simulink model "diva_R2020a"  (R2020a)
settings: Solver=FixedStepDiscrete  StartTime=0.0  StopTime=0.66  RelTol=1e-3  EnableMultiTasking=on
InitFcn:
  | diva_callback_initfcn
StopFcn:
  | diva_callback_stopfcn
undefined symbols (not defined in the file or in its folder): diva_hanning
libraries: simulink x13
CloseFcn:
  | diva_callback_closefcn
settings Model: Creator=alfnie  LastModifiedBy=alfnie
settings DataIOCC: SaveFormat=Array  ReturnWorkspaceOutputs=off
settings OptimizationCC: ExpressionDepthLimit=2147483647  LifeSpan=inf
settings DebuggingCC: UnderspecifiedInitializationDetection=Classic  MergeDetectMultiDrivingBlocksExec=none  SolverPrmCheckMsg=warning  FcnCallInpInsideContextMsg=warning  StateNameClashWarn=warning  SFUnexpectedBacktrackingDiag=warning  SFNoUnconditionalDefaultTransitionDiag=warning  SFExecutionAtInitializationDiag=none  ArithmeticOperatorsInVariantConditions=warning
settings HardwareCC: ProdBitPerPointer=32  ProdBitPerSizeT=32  ProdBitPerPtrDiffT=32  ProdLargestAtomicFloat=None  ProdIntDivRoundTo=Undefined  ProdEndianess=Unspecified  ProdWordSize=32  ProdHWDeviceType=32-bit Generic
settings ModelReferenceCC: PropagateSignalLabelsOutOfModel=off
settings SFSimCC: SimUseLocalCustomCode=off  CustomCodeUndefinedFunction=UseInterfaceOnly
settings RTWCC: RTWUseLocalCustomCode=off
settings CodeAppCC: StateflowObjectComments=on
settings GRTTargetCC: TargetLangStandard=C89/C90 (ANSI)  CombineOutputUpdateFcns=off  GRTInterface=on
settings ConfigComp: CovMetricSettings=dw  CovHtmlReporting=on  CovSaveCumulativeToWorkspaceVar=on  CovSaveSingleToWorkspaceVar=on  CovExternalEMLEnable=off

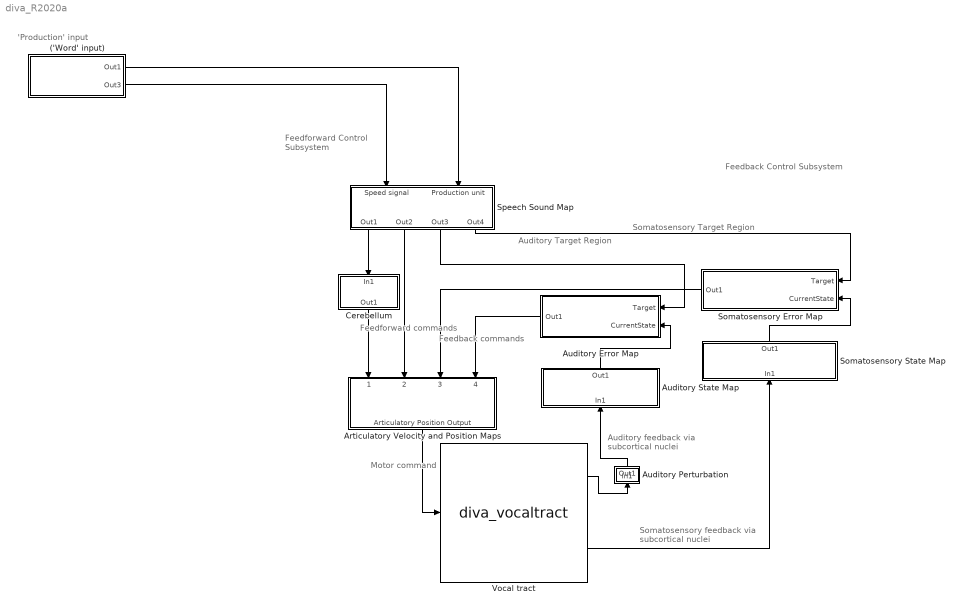
== system diva_R2020a ==
  note: 'Production' input
  note: Feedback Control Subsystem
  note: Somatosensory Target Region
  note: Auditory Target Region
  note: Feedback
      | commands
  note: Feedforward
      | Control
      | Subsystem
  note: Auditory feedback via
      | subcortical nuclei
  note: Somatosensory feedback via
      | subcortical nuclei
  note: Feedforward
      | commands
  note: Motor command
  ('Word' input) : Subsystem
      mask Display:
      | port_label('output',1,'Production unit')
      | port_label('output',2,'GO/speed signal')
  Articulatory Velocity and Position Maps : Subsystem
      mask Display: disp('Articulatory Velocity\newlineand Position Maps\newline{\rm\fontsize{12}\it     (Motor Cortex)}','texmode','on')
  Auditory Error Map : Subsystem
      mask Display: disp('Auditory Error Map\newline{\rm\fontsize{12}\it(Sup. Temporal Cortex)}','texmode','on')
  Auditory Perturbation : Subsystem  mask{perturbationsize=[0,0,0,0], perturbationtime=100, perturbationduration=200}
      mask prompts: perturbationsize "Perturbation size (F0-F3 change in Hz)"; perturbationtime "Perturbation onset (ms)"; perturbationduration "Perturbation duration (ms)"
      mask Display: plot([1,2,2,3,3,4],[0,1,0,1,0,1])
  Auditory State Map : Subsystem
      mask Display: disp('Auditory State Map\newline{\rm\fontsize{12}\it(Sup. Temporal Cortex)}','texmode','on')
  Cerebellum : Subsystem
      mask Display: disp('{\rm\fontsize{12}\itCerebellum}','texmode','on')
  Somatosensory Error Map : Subsystem
      mask Display: disp('Somatosensory Error Map\newline{\rm\fontsize{12}\it       (Inf. Parietal Cortex)}','texmode','on')
  Somatosensory State Map : Subsystem
      mask Display: disp('Somatosensory State Map\newline{\rm\fontsize{12}\it         (Inf. Parietal Cortex)}','texmode','on')
  Speech Sound Map : Subsystem
      mask Display: disp('Speech Sound Map\newline{\rm\fontsize{12}\it(Left Ventral Premotor Cortex)}','texmode','on')
  Vocal tract : M-S-Function  FunctionName=diva_vocaltract
      mask help: Vocal Tract model
      mask Display: image('diva_vocaltract.jpg')
  wires:
  Speech Sound Map/1(Out1) -> Cerebellum/1(In1)
  Auditory State Map/1(Out1) -> Auditory Error Map/2(CurrentState)
  Cerebellum/1(Out1) -> Articulatory Velocity and Position Maps/1(Cerebellum Input)
  Articulatory Velocity and Position Maps/1(Articulatory Position Output) -> Vocal tract/1
  Speech Sound Map/3(Out3) -> Auditory Error Map/1(Target)
  Speech Sound Map/2(Out2) -> Articulatory Velocity and Position Maps/2(SSM Input)
  ('Word' input)/1(Out1) -> Speech Sound Map/2(Production unit)
  ('Word' input)/2(Out3) -> Speech Sound Map/1(Speed signal)
  Speech Sound Map/4(Out4) -> Somatosensory Error Map/1(Target)
  Somatosensory State Map/1(Out1) -> Somatosensory Error Map/2(CurrentState)
  Vocal tract/1 -> Auditory Perturbation/1(In1)
  Vocal tract/2 -> Somatosensory State Map/1(In1)
  Somatosensory Error Map/1(Out1) -> Articulatory Velocity and Position Maps/3(Somatosensory Error Input)
  Auditory Error Map/1(Out1) -> Articulatory Velocity and Position Maps/4(Auditory Error Input)
  Auditory Perturbation/1(Out1) -> Auditory State Map/1(In1)

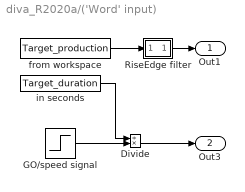
== system diva_R2020a/('Word' input) ==
  Divide : Product  Inputs=/*
  GO/speed signal : Step  Time=0  SampleTime=0
  RiseEdge filter : Subsystem
      mask Display: plot([0,.5,.5,1],[0,0,1,1])
  from workspace : FromWorkspace  VariableName=Target_production  SampleTime=.005  Interpolate=off  OutputAfterFinalValue=Holding final value
  in seconds : FromWorkspace  VariableName=Target_duration  SampleTime=.005  Interpolate=off  OutputAfterFinalValue=Holding final value
  Out1 : Outport
  Out3 : Outport  Port=2
  wires:
  from workspace/1 -> RiseEdge filter/1(In1)
  RiseEdge filter/1(Out1) -> Out1/1
  Divide/1 -> Out3/1
  GO/speed signal/1 -> Divide/2
  in seconds/1 -> Divide/1

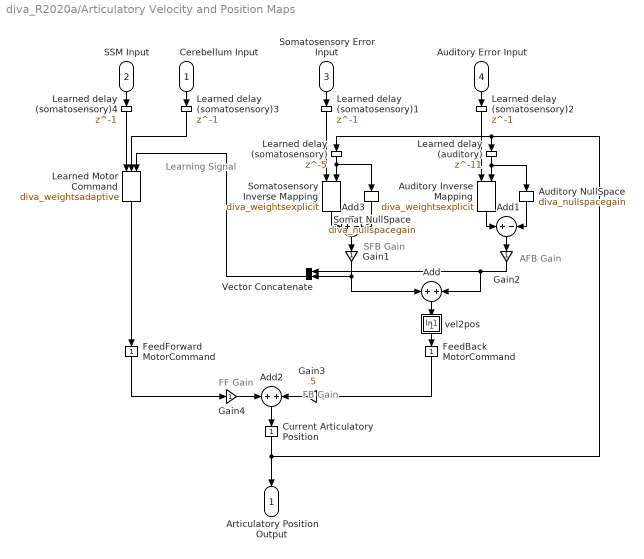
== system diva_R2020a/Articulatory Velocity and Position Maps ==
  note: Learning
      | Signal
  note: FF Gain
  note: FB Gain
  note: SFB Gain
  note: AFB Gain
  Cerebellum Input : Inport
  SSM Input : Inport  Port=2
  Somatosensory Error Input : Inport  Port=3
  Auditory Error Input : Inport  Port=4
  Add : Sum
  Add1 : Sum  Inputs=+-
  Add2 : Sum
  Add3 : Sum  Inputs=+-
  Auditory Inverse Mapping : M-S-Function  FunctionName=diva_weightsexplicit  Parameters=index,epsilon,lambda  mask{index=Auditory, epsilon=.05, lambda=.05}
      mask prompts: index "Vocal Tract output type:"; epsilon "Jacobian step size:"; lambda "Jacobian regularization factor:"
      mask help: Inverse map (explicit computation)
      mask TypeOptions index: Auditory | Somatosensory
      mask Display:
      | plot([0,.50,.50,0.51,0.51,0.60,0.67,0.75,0.75,0.67,0.60,0.51,0.51,0.50],[.5,.5,0.50,0.35,0.21,0.10,0.02,0.00,1.00,0.98,0.90,0.79,0.65,0.50])
      | %patch([0.525 0.533 0.565 0.605 0.661 0.725 0.725 0.661 0.605 0.565 0.533 0.525],[0.5 0.38 0.268 0.18 0.116 0.1 0.9 0.884 0.82 0.732 0.62 0.5],0*[1,1,1])
  Auditory NullSpace : M-S-Function  FunctionName=diva_nullspacegain  Parameters=k,index,epsilon,lambda  mask{k=.10, index=Auditory&Somatosensory, epsilon=.05, lambda=.05}
      mask prompts: k "Gain:"; index "Vocal Tract output type:"; epsilon "Jacobian step size:"; lambda "Jacobian regularization factor:"
      mask help: Null-space projection
      mask TypeOptions index: Auditory | Somatosensory | Auditory&Somatosensory
      mask Display:
      | plot([.2,.2,.8,.2],[.2,.8,.5,.2])
      | disp('\bf~','texmode','on')
  Current Articulatory Position : simulink/Math Operations/Slider Gain  gain=1  low=0  high=2
  FeedBack MotorCommand : simulink/Math Operations/Slider Gain  gain=1  low=0  high=2
  FeedForward MotorCommand : simulink/Math Operations/Slider Gain  gain=1  low=0  high=2
  Gain1 : Gain
  Gain2 : Gain
  Gain3 : Gain  Gain=.5
  Gain4 : Gain
  Learned Motor Command : M-S-Function  FunctionName=diva_weightsadaptive  Parameters=filename,alpha  mask{filename=diva_weights_SSM2FF.mat, alpha=.10}
      mask prompts: filename "Weight Matrix filename:"; alpha "Learning rate:"
      mask help: Adaptive weights
      mask Display:
      | plot([0,.50,.50,0.51,0.51,0.60,0.67,0.75,0.75,0.67,0.60,0.51,0.51,0.50],[.5,.5,0.50,0.35,0.21,0.10,0.02,0.00,1.00,0.98,0.90,0.79,0.65,0.50])
      | %patch(.625+.8*([0.50,0.51,0.55,0.60,0.67,0.75,0.75,0.67,0.60,0.55,0.51,0.50]-.625),.5+.8*([0.50,0.35,0.21,0.10,0.02,0.00,1.00,0.98,0.90,0.79,0.65,0.50]-.5),1*[1,1,1])
      | plot([.2,.4],[.2,.8])
  Learned delay (auditory) : Delay  DelayLength=11  InitialCondition=0
  Learned delay (somatosensory) : Delay  DelayLength=5  InitialCondition=0
  Learned delay (somatosensory){1..4} (4 alike) : Delay  DelayLength=1  InitialCondition=0
  Somat NullSpace : M-S-Function  FunctionName=diva_nullspacegain  Parameters=k,index,epsilon,lambda  mask{k=.10, index=Auditory&Somatosensory, epsilon=.05, lambda=.05}
      mask prompts: k "Gain:"; index "Vocal Tract output type:"; epsilon "Jacobian step size:"; lambda "Jacobian regularization factor:"
      mask help: Null-space projection
      mask TypeOptions index: Auditory | Somatosensory | Auditory&Somatosensory
      mask Display:
      | plot([.2,.2,.8,.2],[.2,.8,.5,.2])
      | disp('\bf~','texmode','on')
  Somatosensory Inverse Mapping : M-S-Function  FunctionName=diva_weightsexplicit  Parameters=index,epsilon,lambda  mask{index=Somatosensory, epsilon=.05, lambda=.05}
      mask prompts: index "Vocal Tract output type:"; epsilon "Jacobian step size:"; lambda "Jacobian regularization factor:"
      mask help: Inverse map (explicit computation)
      mask TypeOptions index: Auditory | Somatosensory
      mask Display:
      | plot([0,.50,.50,0.51,0.51,0.60,0.67,0.75,0.75,0.67,0.60,0.51,0.51,0.50],[.5,.5,0.50,0.35,0.21,0.10,0.02,0.00,1.00,0.98,0.90,0.79,0.65,0.50])
      | %patch(.625+.8*([0.50,0.51,0.55,0.60,0.67,0.75,0.75,0.67,0.60,0.55,0.51,0.50]-.625),.5+.8*([0.50,0.35,0.21,0.10,0.02,0.00,1.00,0.98,0.90,0.79,0.65,0.50]-.5),1*[1,1,1])
  Vector Concatenate : Concatenate
  vel2pos : Subsystem  mask{factor=0.95}
      mask prompts: factor "Integrator factor"
      mask Display: plot([0 .1 .1 .15 nan .4 .35 .35 .4 .4 nan .45 .5 nan .45 .5],[-1 -1 1 1 nan .1 .1 0 0 .5 nan 0 .1 nan .1 0])
  Articulatory Position Output : Outport
  wires:
  Somatosensory Inverse Mapping/1 -> Add3/1
  Add2/1 -> Current Articulatory Position/1
  Current Articulatory Position/1 -> Learned delay (somatosensory)/1, Learned delay (auditory)/1, Articulatory Position Output/1
  SSM Input/1 -> Learned delay (somatosensory)4/1
  Cerebellum Input/1 -> Learned delay (somatosensory)3/1
  Auditory Error Input/1 -> Learned delay (somatosensory)2/1
  Somatosensory Error Input/1 -> Learned delay (somatosensory)1/1
  Gain2/1 -> Add/2, Vector Concatenate/1
  Gain1/1 -> Add/1, Vector Concatenate/2
  Vector Concatenate/1 -> Learned Motor Command/3
  Learned delay (auditory)/1 -> Auditory Inverse Mapping/2, Auditory NullSpace/1
  Learned delay (somatosensory)/1 -> Somat NullSpace/1, Somatosensory Inverse Mapping/2
  Learned delay (somatosensory)1/1 -> Somatosensory Inverse Mapping/1
  Learned delay (somatosensory)2/1 -> Auditory Inverse Mapping/1
  Learned delay (somatosensory)3/1 -> Learned Motor Command/2
  Learned delay (somatosensory)4/1 -> Learned Motor Command/1
  FeedBack MotorCommand/1 -> Gain3/1
  Auditory NullSpace/1 -> Add1/2
  Somat NullSpace/1 -> Add3/2
  Gain3/1 -> Add2/2
  Learned Motor Command/1 -> FeedForward MotorCommand/1
  Gain4/1 -> Add2/1
  Auditory Inverse Mapping/1 -> Add1/1
  Add/1 -> vel2pos/1(In1)
  vel2pos/1(Out1) -> FeedBack MotorCommand/1
  Add3/1 -> Gain1/1
  Add1/1 -> Gain2/1
  FeedForward MotorCommand/1 -> Gain4/1

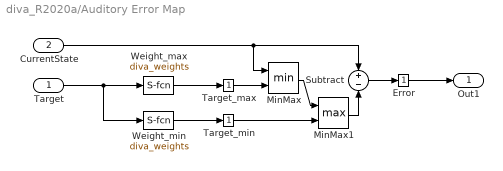
== system diva_R2020a/Auditory Error Map ==
  Target : Inport
  CurrentState : Inport  Port=2
  Error : simulink/Math Operations/Slider Gain  gain=1  low=0  high=2
  MinMax : MinMax  Inputs=2  ZeroCross=off
  MinMax1 : MinMax  Function=max  Inputs=2  ZeroCross=off
  Subtract : Sum  Inputs=+-
  Target_max : simulink/Math Operations/Slider Gain  gain=1  low=0  high=2
  Target_min : simulink/Math Operations/Slider Gain  gain=1  low=0  high=2
  Weight_max : M-S-Function  FunctionName=diva_weights  Parameters=filename  mask{filename=diva_weights_SSM2amax.mat}
      mask prompts: filename "Weight Matrix filename:"
      mask help: Weights
      mask Display:
      | plot([0,.5,0.50,0.51,0.55,0.60,0.67,0.75,0.75,0.67,0.60,0.55,0.51,0.50],[.5,.5,0.50,0.35,0.21,0.10,0.02,0.00,1.00,0.98,0.90,0.79,0.65,0.50])
      | patch(.625+.8*([0.50,0.51,0.55,0.60,0.67,0.75,0.75,0.67,0.60,0.55,0.51,0.50]-.625),.5+.8*([0.50,0.35,0.21,0.10,0.02,0.00,1.00,0.98,0.90,0.79,0.65,0.50]-.5),1*[1,1,1])
  Weight_min : M-S-Function  FunctionName=diva_weights  Parameters=filename  mask{filename=diva_weights_SSM2amin.mat}
      mask prompts: filename "Weight Matrix filename:"
      mask help: Weights
      mask Display:
      | plot([0,.5,0.50,0.51,0.55,0.60,0.67,0.75,0.75,0.67,0.60,0.55,0.51,0.50],[.5,.5,0.50,0.35,0.21,0.10,0.02,0.00,1.00,0.98,0.90,0.79,0.65,0.50])
      | patch(.625+.8*([0.50,0.51,0.55,0.60,0.67,0.75,0.75,0.67,0.60,0.55,0.51,0.50]-.625),.5+.8*([0.50,0.35,0.21,0.10,0.02,0.00,1.00,0.98,0.90,0.79,0.65,0.50]-.5),1*[1,1,1])
  Out1 : Outport
  wires:
  Error/1 -> Out1/1
  Subtract/1 -> Error/1
  Weight_max/1 -> Target_max/1
  MinMax/1 -> MinMax1/1
  Weight_min/1 -> Target_min/1
  Target/1 -> Weight_max/1, Weight_min/1
  CurrentState/1 -> Subtract/1, MinMax/1
  MinMax1/1 -> Subtract/2
  Target_max/1 -> MinMax/2
  Target_min/1 -> MinMax1/2

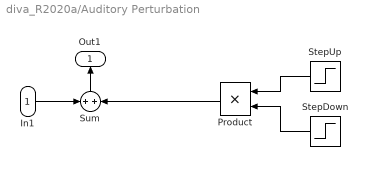
== system diva_R2020a/Auditory Perturbation ==
  In1 : Inport
  Product : Product
  StepDown : Step  Time=perturbationtime/1000+perturbationduration/1000  Before=1  After=0  SampleTime=0
  StepUp : Step  Time=perturbationtime/1000  After=perturbationsize./[100,500,1500,3000]  SampleTime=0
  Sum : Sum
  Out1 : Outport
  wires:
  StepUp/1 -> Product/1
  Sum/1 -> Out1/1
  In1/1 -> Sum/1
  StepDown/1 -> Product/2
  Product/1 -> Sum/2

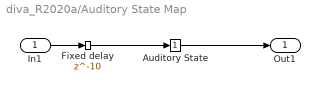
== system diva_R2020a/Auditory State Map ==
  In1 : Inport
  Auditory State : simulink/Math Operations/Slider Gain  gain=1  low=0  high=2
  Fixed delay : Delay  DelayLength=10
  Out1 : Outport
  wires:
  Auditory State/1 -> Out1/1
  In1/1 -> Fixed delay/1
  Fixed delay/1 -> Auditory State/1

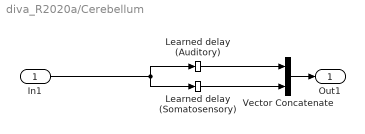
== system diva_R2020a/Cerebellum ==
  In1 : Inport
  Learned delay (Auditory) : DiscreteFir  Coefficients=diva_hanning(11,.5,.95)  AccumDataTypeStr=Inherit: Same as product output
  Learned delay (Somatosensory) : DiscreteFir  Coefficients=diva_hanning(5,.5,.95)  AccumDataTypeStr=Inherit: Same as product output
  Vector Concatenate : Concatenate
  Out1 : Outport
  wires:
  In1/1 -> Learned delay (Somatosensory)/1, Learned delay (Auditory)/1
  Vector Concatenate/1 -> Out1/1
  Learned delay (Auditory)/1 -> Vector Concatenate/1
  Learned delay (Somatosensory)/1 -> Vector Concatenate/2

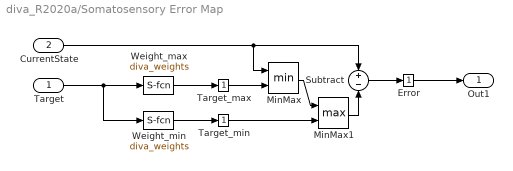
== system diva_R2020a/Somatosensory Error Map ==
  Target : Inport
  CurrentState : Inport  Port=2
  Error : simulink/Math Operations/Slider Gain  gain=1  low=0  high=2
  MinMax : MinMax  Inputs=2  ZeroCross=off
  MinMax1 : MinMax  Function=max  Inputs=2  ZeroCross=off
  Subtract : Sum  Inputs=+-
  Target_max : simulink/Math Operations/Slider Gain  gain=1  low=0  high=2
  Target_min : simulink/Math Operations/Slider Gain  gain=1  low=0  high=2
  Weight_max : M-S-Function  FunctionName=diva_weights  Parameters=filename  mask{filename=diva_weights_SSM2smax.mat}
      mask prompts: filename "Weight Matrix filename:"
      mask help: Weights
      mask Display:
      | plot([0,.5,0.50,0.51,0.55,0.60,0.67,0.75,0.75,0.67,0.60,0.55,0.51,0.50],[.5,.5,0.50,0.35,0.21,0.10,0.02,0.00,1.00,0.98,0.90,0.79,0.65,0.50])
      | patch(.625+.8*([0.50,0.51,0.55,0.60,0.67,0.75,0.75,0.67,0.60,0.55,0.51,0.50]-.625),.5+.8*([0.50,0.35,0.21,0.10,0.02,0.00,1.00,0.98,0.90,0.79,0.65,0.50]-.5),1*[1,1,1])
  Weight_min : M-S-Function  FunctionName=diva_weights  Parameters=filename  mask{filename=diva_weights_SSM2smin.mat}
      mask prompts: filename "Weight Matrix filename:"
      mask help: Weights
      mask Display:
      | plot([0,.5,0.50,0.51,0.55,0.60,0.67,0.75,0.75,0.67,0.60,0.55,0.51,0.50],[.5,.5,0.50,0.35,0.21,0.10,0.02,0.00,1.00,0.98,0.90,0.79,0.65,0.50])
      | patch(.625+.8*([0.50,0.51,0.55,0.60,0.67,0.75,0.75,0.67,0.60,0.55,0.51,0.50]-.625),.5+.8*([0.50,0.35,0.21,0.10,0.02,0.00,1.00,0.98,0.90,0.79,0.65,0.50]-.5),1*[1,1,1])
  Out1 : Outport
  wires:
  Subtract/1 -> Error/1
  CurrentState/1 -> MinMax/1, Subtract/1
  Target/1 -> Weight_max/1, Weight_min/1
  Weight_max/1 -> Target_max/1
  MinMax/1 -> MinMax1/1
  Weight_min/1 -> Target_min/1
  MinMax1/1 -> Subtract/2
  Target_max/1 -> MinMax/2
  Target_min/1 -> MinMax1/2
  Error/1 -> Out1/1

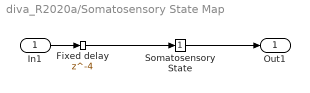
== system diva_R2020a/Somatosensory State Map ==
  In1 : Inport
  Fixed delay : Delay  DelayLength=4
  Somatosensory State : simulink/Math Operations/Slider Gain  gain=1  low=0  high=2
  Out1 : Outport
  wires:
  Somatosensory State/1 -> Out1/1
  In1/1 -> Fixed delay/1
  Fixed delay/1 -> Somatosensory State/1

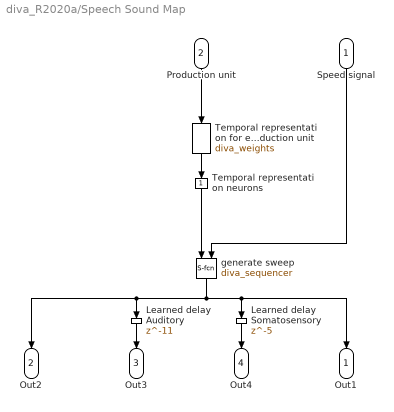
== system diva_R2020a/Speech Sound Map ==
  Speed signal : Inport
  Production unit : Inport  Port=2
  Learned delay Auditory : Delay  DelayLength=11
  Learned delay Somatosensory : Delay  DelayLength=5
  Temporal representation neurons : simulink/Math Operations/Slider Gain  gain=1  low=0  high=2
  Temporal representation for each production unit : M-S-Function  FunctionName=diva_weights  Parameters=filename  mask{filename=diva_weights_SSM.mat}
      mask prompts: filename "Weight Matrix filename:"
      mask help: Weights
      mask Display:
      | plot([0,.5,0.50,0.51,0.55,0.60,0.67,0.75,0.75,0.67,0.60,0.55,0.51,0.50],[.5,.5,0.50,0.35,0.21,0.10,0.02,0.00,1.00,0.98,0.90,0.79,0.65,0.50])
      | patch(.625+.8*([0.50,0.51,0.55,0.60,0.67,0.75,0.75,0.67,0.60,0.55,0.51,0.50]-.625),.5+.8*([0.50,0.35,0.21,0.10,0.02,0.00,1.00,0.98,0.90,0.79,0.65,0.50]-.5),1*[1,1,1])
  generate sweep : M-S-Function  FunctionName=diva_sequencer
      mask Display: plot([1.00, 0.98, 0.92, 0.82, 0.69, 0.53, 0.35, 0.15,-0.05,-0.25,-0.44,-0.61,-0.76,-0.87,-0.95,-0.99,-0.99,-0.95,-0.87,-0.76,-0.61,-0.44,-0.25,-0.05, 0.15, 0.35, 0.53, 0.69, 0.82, 0.92, 0.98, 1.00],[0.00, 0.20, 0.39, 0.57, 0.72, 0.85, 0.94, 0.99, 1.00, 0.97, 0.90, 0.79, 0.65, 0.49, 0.30, 0.10,-0.10,-0.30,-0.49,-0.65,-0.79,-0.90,-0.97,-1.00,-0.99,-0.94,-0.85,-0.72,-0.57,-0.39,-0.20,-0.00])
  Out1 : Outport
  Out2 : Outport  Port=2
  Out3 : Outport  Port=3
  Out4 : Outport  Port=4
  wires:
  Temporal representation for each production unit/1 -> Temporal representation neurons/1
  generate sweep/1 -> Out2/1, Learned delay Auditory/1, Out1/1, Learned delay Somatosensory/1
  Production unit/1 -> Temporal representation for each production unit/1
  Speed signal/1 -> generate sweep/2
  Learned delay Somatosensory/1 -> Out4/1
  Learned delay Auditory/1 -> Out3/1
  Temporal representation neurons/1 -> generate sweep/1

== system diva_R2020a/('Word' input)/RiseEdge filter ==
  In1 : Inport
  DetectRiseFromZero1 : Subsystem
      mask Display: plot([0,.5,.5,1],[0,0,1,1])
  Product1 : Product  RndMeth=Zero
  Out1 : Outport
  wires:
  DetectRiseFromZero1/1(Out1) -> Product1/2
  In1/1 -> DetectRiseFromZero1/1(In1), Product1/1
  Product1/1 -> Out1/1

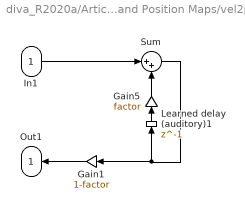
== system diva_R2020a/Articulatory Velocity and Position Maps/vel2pos ==
  In1 : Inport
  Gain1 : Gain  Gain=1-factor
  Gain5 : Gain  Gain=factor
  Learned delay (auditory)1 : Delay  DelayLength=1  InitialCondition=0
  Sum : Sum  Inputs=|++
  Out1 : Outport
  wires:
  In1/1 -> Sum/1
  Gain5/1 -> Sum/2
  Learned delay (auditory)1/1 -> Gain5/1
  Sum/1 -> Gain1/1, Learned delay (auditory)1/1
  Gain1/1 -> Out1/1

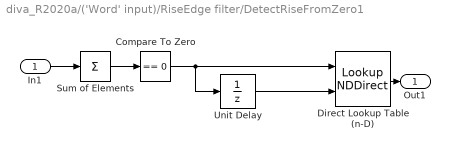
== system diva_R2020a/('Word' input)/RiseEdge filter/DetectRiseFromZero1 ==
  In1 : Inport
  Compare To Zero : simulink/Logic and Bit Operations/Compare To Zero  relop===  OutDataTypeStr=boolean  ZeroCross=off
  Direct Lookup Table (n-D) : LookupNDDirect  Table=[0,1;0,0]
  Sum of Elements : Sum  Inputs=+
  Unit Delay : UnitDelay  InitialCondition=1  SampleTime=-1  HasFrameUpgradeWarning=on
  Out1 : Outport
  wires:
  Direct Lookup Table (n-D)/1 -> Out1/1
  Unit Delay/1 -> Direct Lookup Table (n-D)/2
  Compare To Zero/1 -> Direct Lookup Table (n-D)/1, Unit Delay/1
  In1/1 -> Sum of Elements/1
  Sum of Elements/1 -> Compare To Zero/1
